simulink model "EnergyVerification"  (R2020a)
settings: Solver=VariableStepAuto  StartTime=0.0  StopTime=inf  MaxStep=1e-04  RelTol=1e-3
values from neighbouring files (symbols this model uses):
  DH = [ 0.089    q1     0    pi/2    0     'R' ... (first row only)    [Robot_G18.m]
libraries: vrlib x7, aerolibanimutils x1, dspinverses x1, RobotG18_Blocos x1
settings Model: Creator=Ricardo Henriques  LastModifiedBy=Catarina
settings DataIOCC: ReturnWorkspaceOutputs=off
settings OptimizationCC: LifeSpan=inf
settings DebuggingCC: ArithmeticOperatorsInVariantConditions=warning
settings SFSimCC: SimUseLocalCustomCode=off  CustomCodeUndefinedFunction=UseInterfaceOnly
settings RTWCC: RTWUseLocalCustomCode=off
settings CodeAppCC: StateflowObjectComments=on

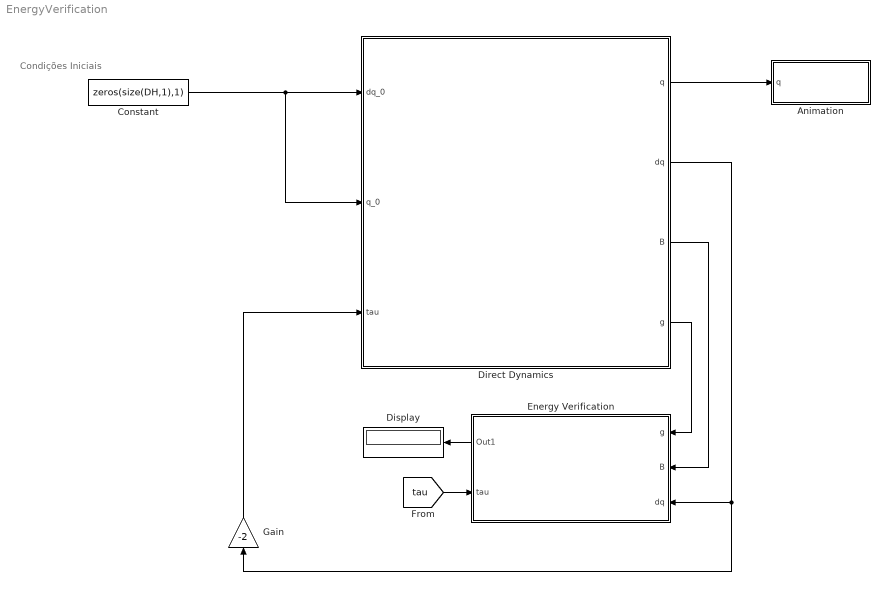
== system EnergyVerification ==
  note: Condições Iniciais
  "Animation " : Subsystem
  Constant : Constant  Value=zeros(size(DH,1),1)  VectorParams1D=off
  Direct Dynamics : Subsystem
  Display : Display
  Energy Verification : Subsystem
      settings: PortSchema="{\"entries\":[{\"content\":{\"sides\":[{\"content\":{\"connectorIds\":[\"In1\",\"In2\",\"In3\"]},\"type\":\"ConnectorPlacement.EquallySpacedRectSide\",\"uuid\":\"4464a4b0-56fe-45bb-a5d3-f20417a48d56\"},{\"content\":{\"connectorIds\":[\"Out1\",\"In4\"],\"side\":\"RIGHT\"},\"type\":\"ConnectorPlacement.EquallySpacedRectSide\",\"uuid\":\"0089294b-f3b6-456d-aaf8-34d4c8861932\"},{\"content\":{\"connectorIds\":[],\"side\":\"TOP\"},\"type\":\"ConnectorPlacement.EquallySpacedRectSide\",\"uuid\":\"f4415ef0-8024-4c43-a982-b53dd61ab6c8\"}]},\"type\":\"ConnectorPlacement.EquallySpacedConnector\",\"uuid\":\"d021274a-5493-4480-88d2-e83904c80acd\"}],\"packageUris\":[\"http://schema.mathworks.com/mf0/Connector/19700101\"],\"version\":\"1.0\"}"
  Gain : Gain  Gain=-2
  wires:
  Energy Verification/1(Out1) -> Display/1
  Direct Dynamics/4(g) -> Energy Verification/1(g)
  Direct Dynamics/3(B) -> Energy Verification/2(B)
  Direct Dynamics/2(dq) -> Energy Verification/3(dq), Gain/1
  Constant/1 -> Direct Dynamics/2(q_0), Direct Dynamics/1(dq_0)
  Direct Dynamics/1(q) -> "Animation "/1("q ")
  [tau] -> Energy Verification/4(tau)
  Gain/1 -> Direct Dynamics/3(tau)

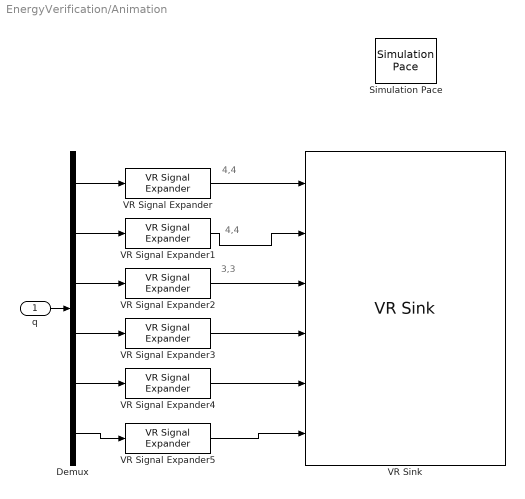
== system EnergyVerification/Animation  ==
  note: 4,4
  note: 3,3
  note: 4,4
  "q " : Inport
  Demux : Demux  Outputs=6
  Simulation Pace : aerolibanimutils/Simulation Pace  SimulationPace=1  SleepMode=Auto  OutputPaceError=off  SampleTime=1/30
  VR Signal Expander{,1..5} (6 alike) : vrlib/VR Signal Expander  outwidth=4  outidx=4
  VR Sink : vrlib/VR Sink  InstantiateOnLoad=on  SampleTime=1/30  ViewEnable=on  RemoteChange=off  RemoteView=off  FieldsWritten=Jt1_DH_dv.rotation.4.1.1.double#Jt2_DH_dv.rotation.4.1.1.double#Jt3_DH_dv.rotation.4.1.1.double#Jt4_DH_dv.rotation.4.1.1.double#Jt5_DH_dv.rotation.4.1.1.double#Jt6_DH_dv.rotation.4.1.1.double  WorldFileName=RobotG18_Opt_NoAxes.wrl  WorldDescription=D-H Reference Frames for Virtual Reality Robot  AutoView=off  VideoDimensions=[]  AllowVariableSize=off  FigureProperties="{'Position', 'Name', 'Viewpoint', 'CameraBound', 'CameraDirection', 'CameraPosition', 'CameraUpVector', 'ZoomFactor', 'Antialiasing', 'Headlight', 'Lighting', 'NavPanel', 'Sound', 'StatusBar', 'Stereo3D', 'Stereo3DCameraOffset', 'Stereo3DHIT', 'ToolBar', 'Textures', 'Transparency', 'Triad', 'Wireframe', 'NavZones', 'NavMode', 'NavSpeed', 'CaptureFileFormat', 'CaptureFileName', 'Record2DCompressMethod', 'Record2DCompressQuality', 'Record2D', 'Record2DFileName', 'Record2DFPS'; [5.0000000000000000e+00   9.2000000000000000e+01   5.7600000000000000e+02   3.5000000000000000e+02], 'D-H Reference Frames for Virtual Reality Robot', 'View 1', 'on', [9.9833416646828169e-02  -2.4616796996452533e-01  -9.6407189539171090e-01], [0.0000000000000000e+00   0.0000000000000000e+00   0.0000000000000000e+00], [0.0000000000000000e+00   9.6891242171064496e-01  -2.4740395925452296e-01], [1.2100000000000002e+00], 'on', 'on', 'on', 'halfbar', 'on', 'on', 'off', [1.0000000149011612e-01], [0.0000000000000000e+00], 'on', 'on', 'on', 'none', 'off', 'off', 'examine', 'normal', 'tif', '%f_anim_%n.tif', 'auto', [7.5000000000000000e+01], 'off', '%f_anim_%n.avi', 'auto'}"
  wires:
  "q "/1 -> Demux/1
  Demux/1 -> VR Signal Expander/1
  Demux/2 -> VR Signal Expander1/1
  Demux/3 -> VR Signal Expander2/1
  Demux/4 -> VR Signal Expander3/1
  Demux/5 -> VR Signal Expander4/1
  Demux/6 -> VR Signal Expander5/1
  VR Signal Expander/1 -> VR Sink/1
  VR Signal Expander1/1 -> VR Sink/2
  VR Signal Expander5/1 -> VR Sink/6
  VR Signal Expander2/1 -> VR Sink/3
  VR Signal Expander3/1 -> VR Sink/4
  VR Signal Expander4/1 -> VR Sink/5

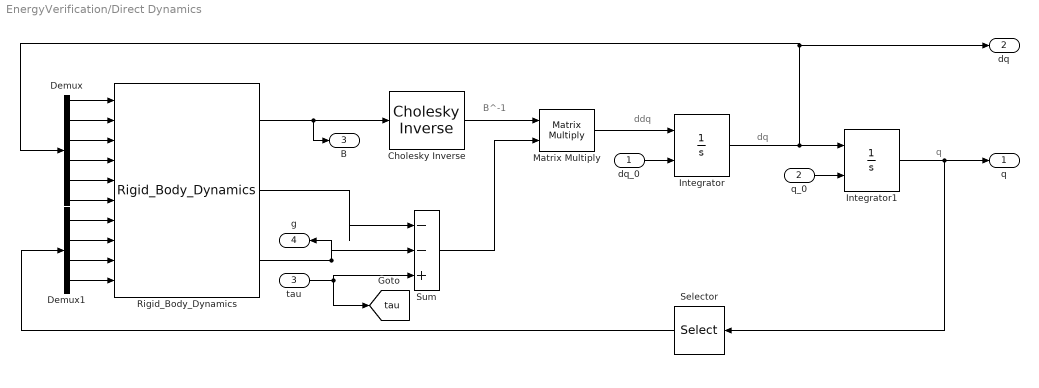
== system EnergyVerification/Direct Dynamics ==
  note: q
  note: dq
  note: ddq
  note: B^-1
  dq_0 : Inport
  q_0 : Inport  Port=2
  tau : Inport  Port=3
  Cholesky Inverse : dspinverses/Cholesky Inverse  errmode=Warning
      settings: SourceProductBaseCode=DS
  Demux : Demux  Outputs=6
  Demux1 : Demux
  Integrator : Integrator  InitialConditionSource=external
  Integrator1 : Integrator  InitialConditionSource=external
  Matrix Multiply : Product  Multiplication=Matrix(*)
  Rigid_Body_Dynamics : RobotG18_Blocos/Rigid_Body_Dynamics  SystemSampleTime=-1  Latency=0  AutoFrameSizeCalculation=off
  Selector : Selector  InputPortWidth=6  IndexOptions=Index vector (dialog)  Indices=[2 3 4 5]  OutputSizes=1
  Sum : Sum  Inputs=|--+
  q : Outport
  dq : Outport  Port=2
  B : Outport  Port=3
  g : Outport  Port=4
  tag scope: tau=global
  wires:
  dq_0/1 -> Integrator/2
  Integrator1/1 -> q/1, Selector/1
  Integrator/1 -> Demux/1, dq/1, Integrator1/1
  q_0/1 -> Integrator1/2
  Matrix Multiply/1 -> Integrator/1
  Cholesky Inverse/1 -> Matrix Multiply/1
  Sum/1 -> Matrix Multiply/2
  Rigid_Body_Dynamics/1 -> B/1, Cholesky Inverse/1
  tau/1 -> [tau], Sum/3
  Rigid_Body_Dynamics/3 -> g/1, Sum/2
  Rigid_Body_Dynamics/2 -> Sum/1
  Demux/1 -> Rigid_Body_Dynamics/1
  Demux/2 -> Rigid_Body_Dynamics/2
  Demux/3 -> Rigid_Body_Dynamics/3
  Demux/4 -> Rigid_Body_Dynamics/4
  Demux/5 -> Rigid_Body_Dynamics/5
  Demux/6 -> Rigid_Body_Dynamics/6
  Demux1/1 -> Rigid_Body_Dynamics/7
  Demux1/2 -> Rigid_Body_Dynamics/8
  Demux1/3 -> Rigid_Body_Dynamics/9
  Demux1/4 -> Rigid_Body_Dynamics/10
  Selector/1 -> Demux1/1

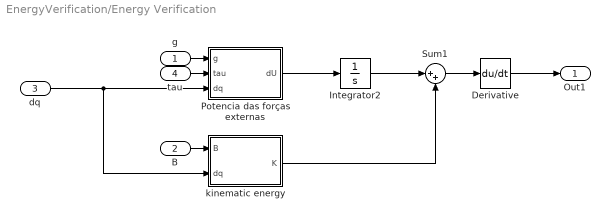
== system EnergyVerification/Energy Verification ==
  g : Inport
  B : Inport  Port=2
  dq : Inport  Port=3
  tau : Inport  Port=4
  Derivative : Derivative
  Integrator2 : Integrator
  Potencia das forças externas : MATLAB Function  TreatAsAtomicUnit=on
  Sum1 : Sum  Inputs=|++
  kinematic energy : MATLAB Function  TreatAsAtomicUnit=on
  Out1 : Outport
  wires:
  Derivative/1 -> Out1/1
  Sum1/1 -> Derivative/1
  dq/1 -> kinematic energy/2(dq), Potencia das forças externas/3(dq)
  tau/1 -> Potencia das forças externas/2(tau)
  Integrator2/1 -> Sum1/1
  g/1 -> Potencia das forças externas/1(g)
  kinematic energy/1(K) -> Sum1/2
  Potencia das forças externas/1(dU) -> Integrator2/1
  B/1 -> kinematic energy/1(B)

== matlab function EnergyVerification/Energy Verification/kinematic energy ==
  data: B input; dq input; K output
function K = kin_en(B,dq)
K = 0.5*dq'*B*dq;
end

== matlab function EnergyVerification/Energy Verification/Potencia das forças externas ==
  data: g input; dU output; tau input; dq input
function dU = work(g,tau,dq)
dU = (g - tau)'*dq;
end
